simulink library "calcDesTanRollAng_ul"  (R2020a)
settings: Solver=VariableStepAuto  StartTime=0.0  StopTime=10.0  RelTol=1e-3
settings Model: Creator=Ayaz  LastModifiedBy=Ayaz

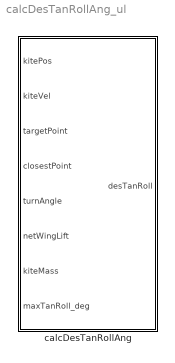
== system calcDesTanRollAng_ul ==
  calcDesTanRollAng : Subsystem

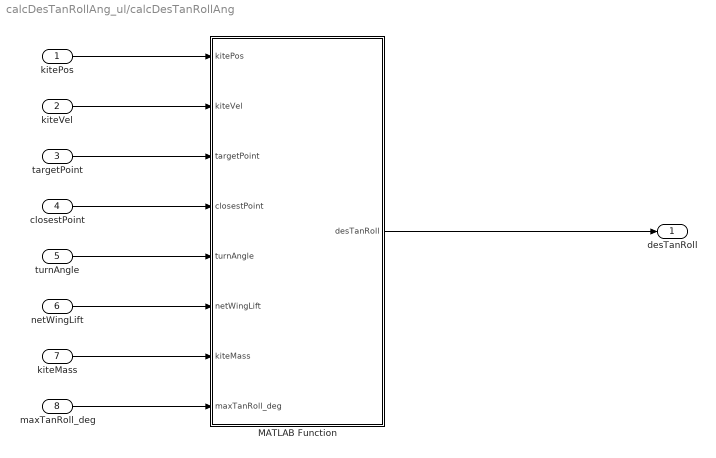
== system calcDesTanRollAng_ul/calcDesTanRollAng ==
  kitePos : Inport
  kiteVel : Inport  Port=2
  targetPoint : Inport  Port=3
  closestPoint : Inport  Port=4
  turnAngle : Inport  Port=5
  netWingLift : Inport  Port=6
  kiteMass : Inport  Port=7
  maxTanRoll_deg : Inport  Port=8
  MATLAB Function : MATLAB Function  TreatAsAtomicUnit=on
  desTanRoll : Outport
  wires:
  targetPoint/1 -> MATLAB Function/3(targetPoint)
  kiteVel/1 -> MATLAB Function/2(kiteVel)
  kitePos/1 -> MATLAB Function/1(kitePos)
  MATLAB Function/1(desTanRoll) -> desTanRoll/1
  maxTanRoll_deg/1 -> MATLAB Function/8(maxTanRoll_deg)
  kiteMass/1 -> MATLAB Function/7(kiteMass)
  netWingLift/1 -> MATLAB Function/6(netWingLift)
  closestPoint/1 -> MATLAB Function/4(closestPoint)
  turnAngle/1 -> MATLAB Function/5(turnAngle)

== matlab function calcDesTanRollAng_ul/calcDesTanRollAng/MATLAB Function ==
  data: kitePos input; desTanRoll output; kiteVel input; targetPoint input; closestPoint input; turnAngle input; netWingLift input; kiteMass input; maxTanRoll_deg input
function desTanRoll = calcDesTanRollAng(kitePos,kiteVel,...
    targetPoint,closestPoint,turnAngle,netWingLift,kiteMass,maxTanRoll_deg)


 desTanRoll = calcDesTanRollAng(kitePos,kiteVel,...
    targetPoint,closestPoint,turnAngle,netWingLift,kiteMass,maxTanRoll_deg);


end
